simulink model "qrotor_system"  (R2022a)
settings: Solver=VariableStepAuto  StartTime=0.0  StopTime=4  RelTol=1e-9
values from neighbouring files (symbols this model uses):
  K = lqr(A,B,Q,R,0)    [controllerLinearizedSystemScript.m]
  testThrust = 0.1    [param.m]    (also in testparam.m = 4)
  testTorque = [0 0 0.1]    [param.m]    (also in testparam.m = [0 0.0001 0])
libraries: matrix_library x1
settings Model: Creator=carlossilvestre  LastModifiedBy=FLKU
settings SolverCC: AlgebraicLoopSolver=TrustRegion
settings DebuggingCC: UnconnectedInputMsg=warning  UnconnectedOutputMsg=warning  UnconnectedLineMsg=warning  SFMachineParentedDataDiag=warning

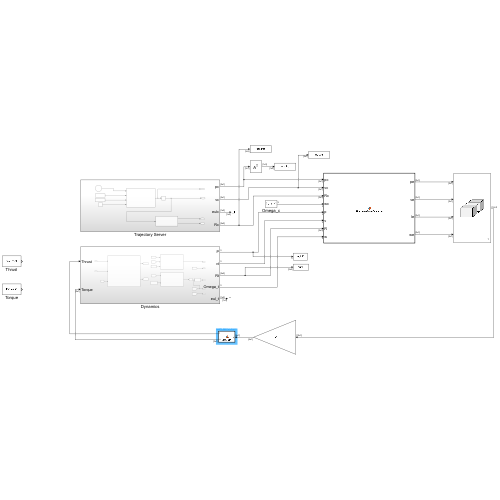
[thumbnail: Simulink's stored preview of the top-level diagram]
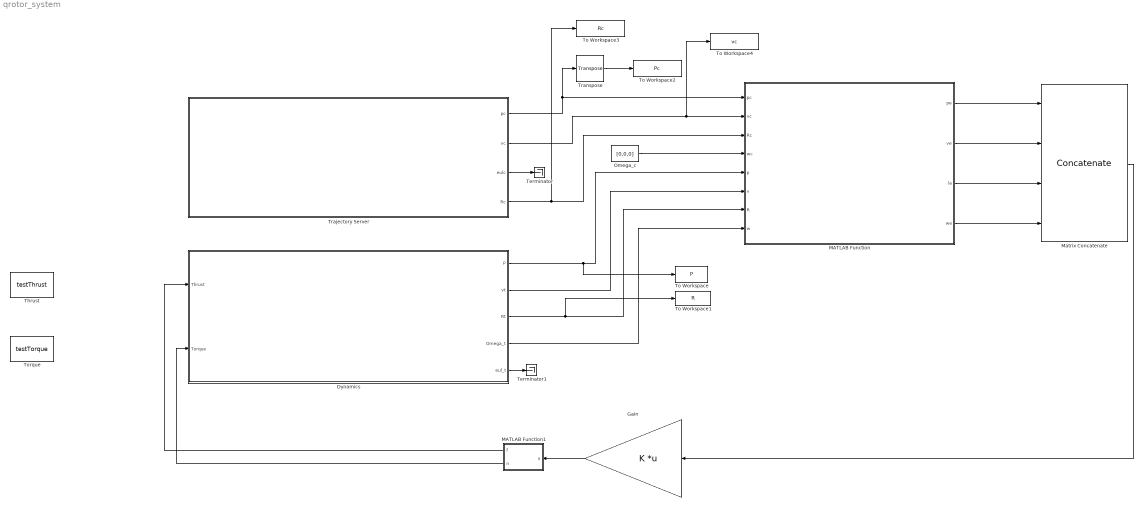
== system qrotor_system ==
  Dynamics : Subsystem
  Gain : Gain  Gain=K  Multiplication=Matrix(K*u)
  MATLAB Function : MATLAB Function  TreatAsAtomicUnit=on
  MATLAB Function1 : MATLAB Function  TreatAsAtomicUnit=on
  Matrix Concatenate : Concatenate  NumInputs=4  Mode=Multidimensional array
  Omega_c : Constant  Value=[0,0,0]
  Terminator : Terminator
  Terminator1 : Terminator
  Thrust : Constant  Value=testThrust
  To Workspace : ToWorkspace  VariableName=P  SaveFormat=Timeseries  SampleTime=-1
  To Workspace1 : ToWorkspace  VariableName=R  SaveFormat=Timeseries  SampleTime=-1
  To Workspace2 : ToWorkspace  VariableName=Pc  SaveFormat=Timeseries  SampleTime=-1
  To Workspace3 : ToWorkspace  VariableName=Rc  SaveFormat=Timeseries  SampleTime=-1
  To Workspace4 : ToWorkspace  VariableName=vc  SaveFormat=Timeseries  SampleTime=-1
  Torque : Constant  Value=testTorque
  Trajectory Server : Subsystem
  Transpose : matrix_library/Transpose
      settings: SourceProductBaseCode=SL
  wires:
  Dynamics/3(Rt) -> To Workspace1/1, MATLAB Function/7(R)
  Dynamics/1(P) -> To Workspace/1, MATLAB Function/5(p)
  Trajectory Server/1(pc) -> Transpose/1, MATLAB Function/1(pc)
  Trajectory Server/2(vc) -> To Workspace4/1, MATLAB Function/2(vc)
  Omega_c/1 -> MATLAB Function/4(wc)
  Dynamics/2(vt) -> MATLAB Function/6(v)
  Dynamics/4(Omega_t) -> MATLAB Function/8(w)
  Trajectory Server/3(eulc) -> Terminator/1
  Trajectory Server/4(Rc) -> To Workspace3/1, MATLAB Function/3(Rc)
  Dynamics/5(eul_t) -> Terminator1/1
  Transpose/1 -> To Workspace2/1
  MATLAB Function/2(ve) -> Matrix Concatenate/2
  MATLAB Function/1(pe) -> Matrix Concatenate/1
  MATLAB Function/3(le) -> Matrix Concatenate/3
  MATLAB Function/4(we) -> Matrix Concatenate/4
  Matrix Concatenate/1 -> Gain/1
  Gain/1 -> MATLAB Function1/1(u)
  MATLAB Function1/1(f) -> Dynamics/1(Thrust)
  MATLAB Function1/2(n) -> Dynamics/2(Torque)

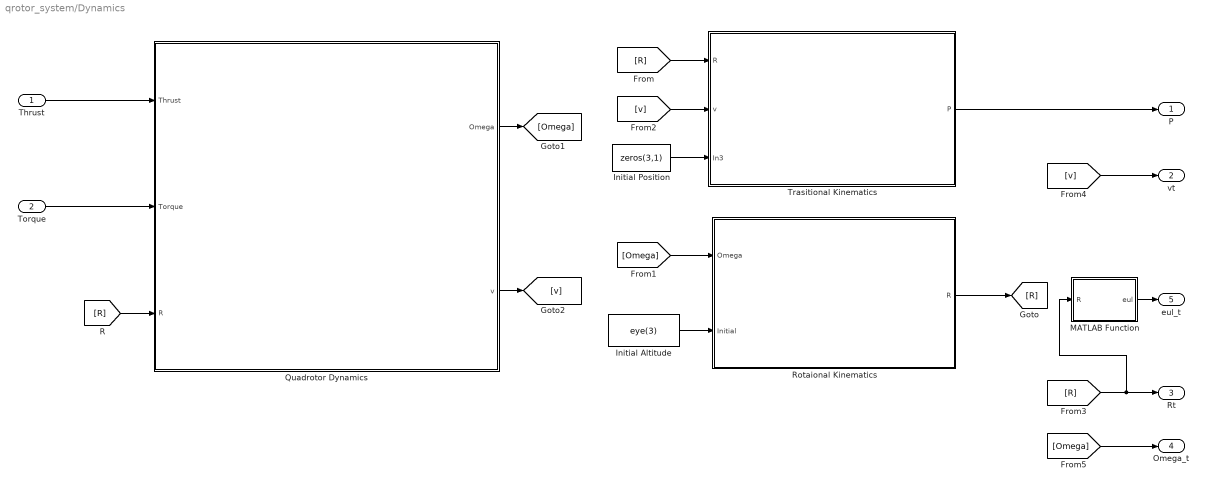
== system qrotor_system/Dynamics ==
  Thrust : Inport
  Torque : Inport  Port=2
  Initial Altitude : Constant  Value=eye(3)
  Initial Position : Constant  Value=zeros(3,1)
  MATLAB Function : MATLAB Function  TreatAsAtomicUnit=on
  Quadrotor Dynamics : Subsystem
  Rotaional Kinematics : Subsystem
  Trasitional Kinematics : Subsystem
  P : Outport
  vt : Outport  Port=2
  Rt : Outport  Port=3
  Omega_t : Outport  Port=4
  eul_t : Outport  Port=5
  wires:
  Quadrotor Dynamics/1(Omega) -> [Omega]
  [R] -> Trasitional Kinematics/1(R)
  Torque/1 -> Quadrotor Dynamics/2(Torque)
  [Omega] -> Rotaional Kinematics/1(Omega)
  [v] -> Trasitional Kinematics/2(v)
  [R] -> Quadrotor Dynamics/3(R)
  Rotaional Kinematics/1(R) -> [R]
  Initial Position/1 -> Trasitional Kinematics/3(In3)
  Initial Altitude/1 -> Rotaional Kinematics/2(Initial)
  Quadrotor Dynamics/2(v) -> [v]
  Thrust/1 -> Quadrotor Dynamics/1(Thrust)
  [R] -> Rt/1, MATLAB Function/1(R)
  Trasitional Kinematics/1(P) -> P/1
  [v] -> vt/1
  [Omega] -> Omega_t/1
  MATLAB Function/1(eul) -> eul_t/1

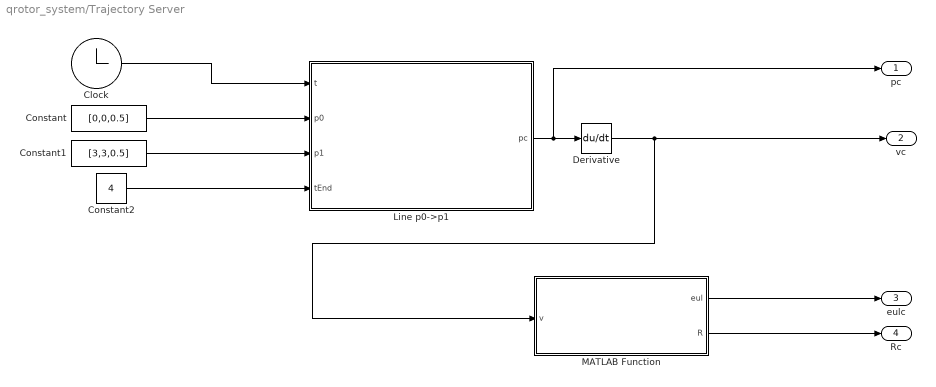
== system qrotor_system/Trajectory Server ==
  Clock : Clock
  Constant : Constant  Value=[0,0,0.5]
  Constant1 : Constant  Value=[3,3,0.5]
  Constant2 : Constant  Value=4
  Derivative : Derivative  CoefficientInTFapproximation=1
  Line p0->p1 : MATLAB Function  TreatAsAtomicUnit=on
  MATLAB Function : MATLAB Function  TreatAsAtomicUnit=on
  pc : Outport
  vc : Outport  Port=2
  eulc : Outport  Port=3
  Rc : Outport  Port=4
  wires:
  Constant2/1 -> Line p0->p1/4(tEnd)
  Constant1/1 -> Line p0->p1/3(p1)
  MATLAB Function/2(R) -> Rc/1
  Derivative/1 -> MATLAB Function/1(v), vc/1
  Clock/1 -> Line p0->p1/1(t)
  Line p0->p1/1(pc) -> pc/1, Derivative/1
  Constant/1 -> Line p0->p1/2(p0)
  MATLAB Function/1(eul) -> eulc/1

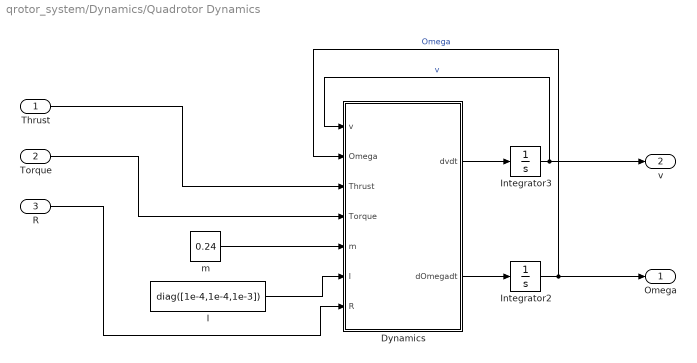
== system qrotor_system/Dynamics/Quadrotor Dynamics ==
  Thrust : Inport
  Torque : Inport  Port=2
  R : Inport  Port=3
  Dynamics : MATLAB Function  TreatAsAtomicUnit=on
  I : Constant  Value=diag([1e-4,1e-4,1e-3])
  Integrator2 : Integrator  InitialCondition=[0,0,0]  ContinuousStateAttributes='omega'
  Integrator3 : Integrator  InitialCondition=[0,0,0]  ContinuousStateAttributes='velocity'
  m : Constant  Value=0.24
  Omega : Outport
  v : Outport  Port=2
  wires:
  Dynamics/1(dvdt) -> Integrator3/1
  Integrator3/1 -> v/1, Dynamics/1(v)  "v"
  R/1 -> Dynamics/7(R)
  Torque/1 -> Dynamics/4(Torque)
  Dynamics/2(dOmegadt) -> Integrator2/1
  I/1 -> Dynamics/6(I)
  Integrator2/1 -> Dynamics/2(Omega), Omega/1  "Omega"
  m/1 -> Dynamics/5(m)
  Thrust/1 -> Dynamics/3(Thrust)

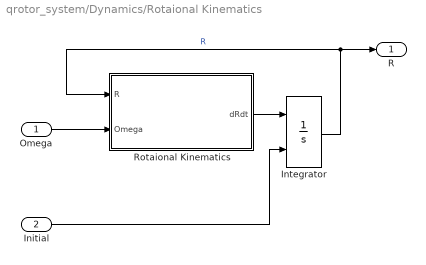
== system qrotor_system/Dynamics/Rotaional Kinematics ==
  Omega : Inport
  Initial : Inport  Port=2
  Integrator : Integrator  InitialConditionSource=external  InitialCondition=eye(3)
  Rotaional Kinematics : MATLAB Function  TreatAsAtomicUnit=on
  R : Outport
  wires:
  Integrator/1 -> Rotaional Kinematics/1(R), R/1  "R"
  Omega/1 -> Rotaional Kinematics/2(Omega)
  Rotaional Kinematics/1(dRdt) -> Integrator/1
  Initial/1 -> Integrator/2

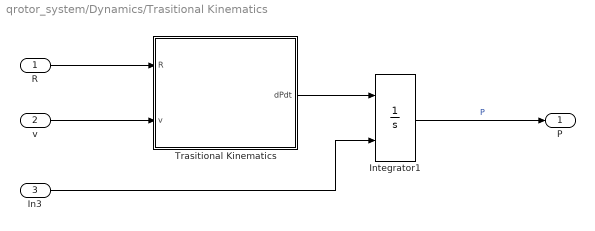
== system qrotor_system/Dynamics/Trasitional Kinematics ==
  R : Inport
  v : Inport  Port=2
  In3 : Inport  Port=3
  Integrator1 : Integrator  InitialConditionSource=external  InitialCondition=[0,0,0]
  Trasitional Kinematics : MATLAB Function  TreatAsAtomicUnit=on
  P : Outport
  wires:
  Integrator1/1 -> P/1  "P"
  Trasitional Kinematics/1(dPdt) -> Integrator1/1
  v/1 -> Trasitional Kinematics/2(v)
  R/1 -> Trasitional Kinematics/1(R)
  In3/1 -> Integrator1/2

== matlab function qrotor_system/Dynamics/Trasitional Kinematics/Trasitional Kinematics ==
  data: R input; dPdt output; v input
function dPdt = CompdPdt(R,v)
dPdt=R*v;
end

== matlab function qrotor_system/Dynamics/Rotaional Kinematics/Rotaional Kinematics ==
  data: R input; dRdt output; Omega input
function dRdt = CompdRdt(R,Omega)
dRdt=R*skew(Omega);
end

== matlab function qrotor_system/Dynamics/Quadrotor Dynamics/Dynamics ==
  data: v input; Omega input; Thrust input; dvdt output; Torque input; dOmegadt output; m input; I input; R input
function [dvdt,dOmegadt] = QDyanamics(v,Omega,Thrust,Torque,m,I,R)
% Quadrotor Dynamics, in quadrotor body coordinate {B}, unless explicitly
% declared.

% m=0.1;
% I=eye(3) * 0.1;
g_scalar = 0;
g_Inertia = [0;0;1] * g_scalar;
g_Body = transpose(R) * g_Inertia;
Force = g_Body + [0;0;-Thrust];
dvdt=-skew(Omega)*v + 1/m*Force;
dOmegadt=-(I^-1)*skew(Omega)*I*Omega + (I^-1)*Torque;
end

== matlab function qrotor_system/Trajectory Server/Line p0->p1 ==
  data: t input; pc output; p0 input; p1 input; tEnd input
function pc = genTraj(t, p0, p1, tEnd)
e = p1-p0;
if t< tEnd
    pc = p0 + t/tEnd * e;
else
    pc = p1;
end
end

== matlab function qrotor_system/Trajectory Server/MATLAB Function ==
  data: v input; eul output; R output
function [eul, R] = genAltitude(v)

z = [0;0;1];
y = cross(z,v);
y = y;
zc = cross(v,y);
z = dot(z,zc) / dot(zc,zc) * zc;
R = [v,y,z];
R = normColVec(R);
eul =rotm2eul(R);

== matlab function qrotor_system/MATLAB Function ==
  data: pc input; pe output; vc input; Rc input; wc input; p input; v input; R input; w input; ve output; le output; we output
function [pe,ve,le,we] = NonLinearTransformation(pc,vc,Rc,wc,p,v,R,w)
pe = transpose(R)*(p-pc);
ve = v-vc;
Re = R*transpose(Rc);
le = transpose(rotm2eul(Re));
we = w-wc;
end

== matlab function qrotor_system/Dynamics/MATLAB Function ==
  data: R input; eul output
function eul = tfR2eul(R)
eul = rotm2eul(R);

== matlab function qrotor_system/MATLAB Function1 ==
  data: u input; f output; n output
function [f,n] = deposite(u)
if max(isnan(u),[],'all')
    u = zeros(4,1);
end
f = u(1);
n = u(2:4);
end
